simulink model "NLKSF"  (Simulink 3.00)
settings: Solver=ode45  SolverMode=SingleTasking  StartTime=0.0  StopTime=40  MaxStep=.025  RelTol=1e-3  AbsTol=1e-3
undefined symbols (not defined in the file or in its folder): h
libraries: simulink3 x1
settings Model: TimeSaveName=t  SaveOutput=off  Creator=CAMPA

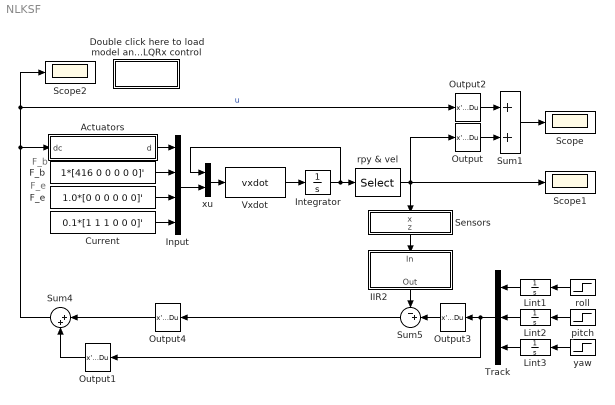
== system NLKSF ==
  note: F_e
  note: F_b
  Actuators : Subsystem
  Current : Constant  Value=0.1*[1 1 1 0 0 0]'
  "Double click here to load model and  LQRx control " : Subsystem
      settings: OpenFcn=shark;h=0.3;global veh;[v1,veh,v3]=vehicle;load abcdk
      mask Display: disp('Load Data')
  F_b : Constant  Value=1*[416 0 0 0 0 0]'
  F_e : Constant  Value=1.0*[0 0 0 0 0 0]'
  IIR2 : Subsystem  Orientation=down  mask(Discrete Time Second Order IIR){ni=9, w=20, x=0.74, x0=0, T=0.025}
      mask prompts: ni "Number of Channels"; w "Poles Magnitude (m)"; x "Poles Damping (x)"; x0 "Initial Condition"; T "Sample Time"
      mask help:
      | Each channel has the transfer function :
      |   1-2*cos(sqrt(1-x^2)*m*T)*exp(-x*m*T)+exp(-2*x*m*T) /
      |   1-2*cos(sqrt(1-x^2)*m*T)*exp(-x*m*T)z^-1+exp(-2*x*m*T)z^-2
      |   which is a good (pz-matched) approximation of
      |   m^2/(s^2+2xms+m^2) if 10*m*T<pi
      |   The initial condition is in discrete time for the whole system.
      mask init:
      | A=[];B=[];C=[];D=[];
      | for i=1:ni,
      | A=[A,zeros(size(A,1),2);zeros(2,size(A,2)),[0 1; -exp(-2*x*w*T) 2*cos(sqrt(1-x^2)*w*T)*exp(-x*w*T)]];
      | B=[B,zeros(size(B,1),1);zeros(2,size(B,2)),[0;1+exp(-2*x*w*T)-2*cos(sqrt(1-x^2)*w*T)*exp(-x*w*T)]];
      | C=[C,zeros(size(C,1),2);zeros(1,size(C,2)),[-exp(-2*x*w*T)  2*cos(sqrt(1-x^2)*w*T)*exp(-x*w*T)]];
      | D=[D,zeros(size(D,1),1);zeros(1,size(D,2)),1+exp(-2*x*w*T)-2*cos(sqrt(1-x^2)*w*T)*exp(-x*w*T)];
      | end
      mask Help:
      | <p>
      |   Each channel has the transfer function :
      |   1-2*cos(sqrt(1-x^2)*m*T)*exp(-x*m*T)+exp(-2*x*m*T) /
      |   1-2*cos(sqrt(1-x^2)*m*T)*exp(-x*m*T)z^-1+exp(-2*x*m*T)z^-2
      |   which is a good (pz-matched) approximation of
      |   m^2/(s^2+2xms+m^2) if 10*m*T<pi
      |   The initial condition is in discrete time for the whole system.
      | </p>
      mask Display: dpoly(w^2, [1 2*x*w w^2],'s')
  Input : Mux  Inputs=[8 6 6 6]
  Integrator : Integrator  ExternalReset=none  InitialConditionSource=internal  InitialCondition=[zeros(6,1);3;zeros(5,1)]  LimitOutput=off  UpperSaturationLimit=inf  LowerSaturationLimit=-inf  ShowSaturationPort=off  ShowStatePort=off  AbsoluteTolerance=auto
  Lint1 : Integrator  Orientation=left  ExternalReset=none  InitialConditionSource=internal  InitialCondition=0  LimitOutput=on  UpperSaturationLimit=h  LowerSaturationLimit=-h  ShowSaturationPort=off  ShowStatePort=off  AbsoluteTolerance=auto
  Lint2 : Integrator  Orientation=left  ExternalReset=none  InitialConditionSource=internal  InitialCondition=0  LimitOutput=on  UpperSaturationLimit=h  LowerSaturationLimit=-h  ShowSaturationPort=off  ShowStatePort=off  AbsoluteTolerance=auto
  Lint3 : Integrator  Orientation=left  ExternalReset=none  InitialConditionSource=internal  InitialCondition=0  LimitOutput=on  UpperSaturationLimit=h  LowerSaturationLimit=-h  ShowSaturationPort=off  ShowStatePort=off  AbsoluteTolerance=auto
  Output : StateSpace  A=[]  B=[]  C=[]  D=K  X0=0  mask(Matrix Gain){@1=c}
      mask prompts: @1 "Gain matrix:"
      mask help: Matrix Gain.
      mask init:
      | K = @1;
      mask Help: Multiplies input vector by entered matrix to produce output vector (y=Au).
      mask Display: disp('C')
  Output1 : StateSpace  Orientation=left  A=[]  B=[]  C=[]  D=K  X0=0  mask(Matrix Gain){@1=pinv(d-c*pinv(a)*b)}
      mask prompts: @1 "Gain matrix:"
      mask help: Matrix Gain.
      mask init:
      | K = @1;
      mask Help: Multiplies input vector by entered matrix to produce output vector (y=Au).
      mask Display: disp('Kf2')
  Output2 : StateSpace  A=[]  B=[]  C=[]  D=K  X0=0  mask(Matrix Gain){@1=d}
      mask prompts: @1 "Gain matrix:"
      mask help: Matrix Gain.
      mask init:
      | K = @1;
      mask Help: Multiplies input vector by entered matrix to produce output vector (y=Au).
      mask Display: disp('D')
  Output3 : StateSpace  Orientation=left  A=[]  B=[]  C=[]  D=K  X0=0  mask(Matrix Gain){@1=eye(9,3)}
      mask prompts: @1 "Gain matrix:"
      mask help: Matrix Gain.
      mask init:
      | K = @1;
      mask Help: Multiplies input vector by entered matrix to produce output vector (y=Au).
      mask Display: disp('Kf1')
  Output4 : StateSpace  Orientation=left  A=[]  B=[]  C=[]  D=K  X0=0  mask(Matrix Gain){@1=K}
      mask prompts: @1 "Gain matrix:"
      mask help: Matrix Gain.
      mask init:
      | K = @1;
      mask Help: Multiplies input vector by entered matrix to produce output vector (y=Au).
      mask Display: disp('K')
  Scope : Scope
      settings: TickLabels=off  TimeRange=40  YMin=-1  YMax=1  SaveName=y  DataFormat=Structure
  Scope1 : Scope
      settings: TickLabels=off  TimeRange=40  YMin=-1  YMax=1  SaveName=x  DataFormat=Structure
  Scope2 : Scope
      settings: TickLabels=off  TimeRange=40  YMin=-1  YMax=1  SaveName=u  DataFormat=Structure
  Sensors : Subsystem  Orientation=down
  Sum1 : Sum  Inputs=++  SaturateOnIntegerOverflow=on
  Sum4 : Sum  Orientation=left  Inputs=|++  SaturateOnIntegerOverflow=on
  Sum5 : Sum  Orientation=left  Inputs=-+|  SaturateOnIntegerOverflow=on
  Track : Mux  Orientation=left  Inputs=3
  Vxdot : MATLABFcn  MATLABFcn=vxdot  OutputWidth=12  OutputSignalType=real
  pitch : Step  Orientation=left  Time=10  Before=0  After=0.1  SampleTime=.1
  roll : Step  Orientation=left  Time=15  Before=0  After=0.1  SampleTime=.1
  rpy & vel : Selector  Elements=[4:12]  InputPortWidth=12
  xu : Mux  Inputs=[12 26]
  yaw : Step  Orientation=left  Time=5  Before=0  After=0.1  SampleTime=.1
  wires:
  Current/1 -> Input/4
  F_b/1 -> Input/2
  F_e/1 -> Input/3
  Actuators/1(d) -> Input/1
  Input/1 -> xu/2
  xu/1 -> Vxdot/1
  Vxdot/1 -> Integrator/1
  Integrator/1 -> xu/1, rpy & vel/1
  Sum4/1 -> Output2/1, Scope2/1, Actuators/1(dc)  "u"
  Sensors/1(z) -> IIR2/1(In)
  Lint1/1 -> Track/1
  IIR2/1(Out) -> Sum5/1
  rpy & vel/1 -> Sensors/1(x), Scope1/1, Output/1
  Sum1/1 -> Scope/1
  Output2/1 -> Sum1/1
  Output/1 -> Sum1/2
  Output4/1 -> Sum4/1
  Output1/1 -> Sum4/2
  Sum5/1 -> Output4/1
  pitch/1 -> Lint2/1
  yaw/1 -> Lint3/1
  Lint2/1 -> Track/2
  Lint3/1 -> Track/3
  Output3/1 -> Sum5/2
  roll/1 -> Lint1/1
  Track/1 -> Output3/1, Output1/1

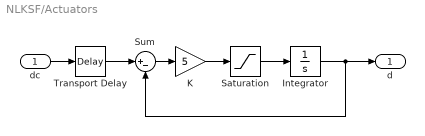
== system NLKSF/Actuators ==
  dc : Inport  Port=1  PortWidth=-1  SampleTime=-1  DataType=auto
      settings: SignalType=auto
  Integrator : Integrator  ExternalReset=none  InitialConditionSource=internal  InitialCondition=0  LimitOutput=on  UpperSaturationLimit=+0.4  LowerSaturationLimit=-0.4  ShowSaturationPort=off  ShowStatePort=off  AbsoluteTolerance=auto
  K : Gain  Gain=5  SaturateOnIntegerOverflow=on
  Saturation : Saturate  UpperLimit=2  LowerLimit=-2
  Sum : Sum  Inputs=|+-  SaturateOnIntegerOverflow=on
  Transport Delay : TransportDelay  DelayTime=0.01  InitialInput=0  BufferSize=2048
  d : Outport  Port=1
  wires:
  Transport Delay/1 -> Sum/1
  dc/1 -> Transport Delay/1
  Saturation/1 -> Integrator/1
  Sum/1 -> K/1
  K/1 -> Saturation/1
  Integrator/1 -> Sum/2, d/1

== system NLKSF/Double click here to load model and  LQRx control  ==

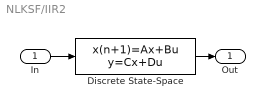
== system NLKSF/IIR2 ==
  In : Inport  Port=1  PortWidth=-1  SampleTime=-1  DataType=auto
      settings: SignalType=auto
  Discrete State-Space : DiscreteStateSpace  A=A  B=B  C=C  D=D  X0=x0  SampleTime=T
  Out : Outport  Port=1
  wires:
  In/1 -> Discrete State-Space/1
  Discrete State-Space/1 -> Out/1

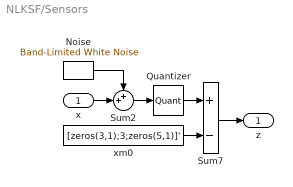
== system NLKSF/Sensors ==
  x : Inport  Port=1  PortWidth=-1  SampleTime=-1  DataType=auto
      settings: SignalType=auto
  Noise : simulink3/Sources/Band-Limited White Noise  Cov=1e-6*ones(1,9)  Ts=0.025  seed=1:9
  Quantizer : Quantizer  QuantizationInterval=0.01
  Sum2 : Sum  Inputs=++|  SaturateOnIntegerOverflow=on
  Sum7 : Sum  Inputs=+-  SaturateOnIntegerOverflow=on
  xm0 : Constant  Value=[zeros(3,1);3;zeros(5,1)]'
  z : Outport  Port=1
  wires:
  x/1 -> Sum2/2
  Sum7/1 -> z/1
  xm0/1 -> Sum7/2
  Sum2/1 -> Quantizer/1
  Quantizer/1 -> Sum7/1
  Noise/1 -> Sum2/1
